simulink model "L2L_HX_test"  (R2014b)
settings: Solver=ode23tb  StartTime=0.0  StopTime=100  RelTol=1e-3
libraries: DAEMOT_Lib x9
settings Model: Creator=pangbor2  LastModifiedBy=koeln2

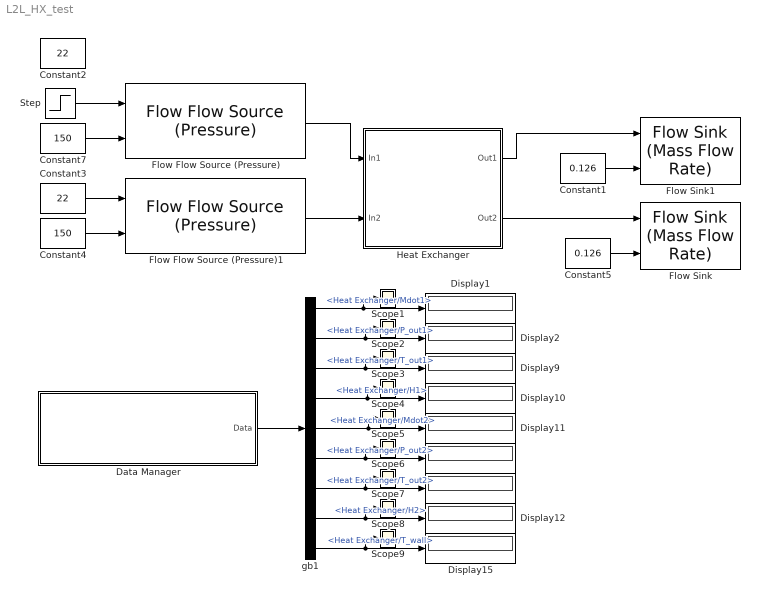
== system L2L_HX_test ==
  "  " : Display
  "   " : Display
  Constant1 : Constant  Value=0.126
  Constant2 : Constant  Value=22
  Constant3 : Constant  Value=22
  Constant4 : Constant  Value=150
  Constant5 : Constant  Value=0.126
  Constant7 : Constant  Value=150
  Data Manager : Subsystem  AncestorBlock=DAEMOT_Lib/Support Functions/Data Manager  mask{null=0}
      mask init:
      | set_param(gcb, 'LinkStatus', 'inactive')    % disable the library link
      settings: OpenFcn=data_manager
      mask Display: str ='Heat Exchanger/Mdot1\nHeat Exchanger/P_out1\nHeat Exchanger/T_out1\nHeat Exchanger/H1\nHeat Exchanger/Mdot2\nHeat Exchanger/P_out2\nHeat Exchanger/T_out2\nHeat Exchanger/H2\nHeat Exchanger/T_wall'; fprintf(str)
  Display{1..2,9..12,15} (7 alike) : Display
  Flow Flow Source (Pressure) : DAEMOT_Lib/Components/Flow Flow Source (Pressure)  M_ext=on  M=0  T_ext=on  T=0  P_ext=on  P=0
  Flow Flow Source (Pressure)1 : DAEMOT_Lib/Components/Flow Flow Source (Pressure)  M_ext=on  M=0  T_ext=on  T=0  P_ext=on  P=0
  Flow Sink : DAEMOT_Lib/Components/Flow Sink (Mass Flow Rate)  M_ext=on  M=0  T_ext=on  T=0  P_ext=on  P=0
  Flow Sink1 : DAEMOT_Lib/Components/Flow Sink (Mass Flow Rate)  M_ext=on  M=0  T_ext=on  T=0  P_ext=on  P=0
  Heat Exchanger : Subsystem  AncestorBlock=DAEMOT_Lib/Components/Heat Exchanger  mask(Heat Exchanger){Tw_init=22, fld1=PG50, P1_init=110, T1_init=22, f1=2, KL1=0, fld2=PG50, P2_init=110, T2_init=22, f2=2, KL2=0, M_wall=1, Cp_wall=0.9, Pass1=6, b1=1*1e-3, W1=87*1e-3, L1=0.193, e1=0.0015*1e-3, Nu_lam1=5.6153, Pass2=6, b2=1*1e-3, W2=87*1e-3, L2=0.193, e2=0.0015*1e-3, Nu_lam2=5.6153}
      mask prompts: Tw_init "Initial Wall Temperature [°C]"; fld1 "Fluid Type 1"; P1_init "Initial Outlet 1 Pressure [kPa]"; T1_init "Initial Outlet 1 Temperature [°C]"; f1 "Friction Factor [-]"; KL1 "Minor Losses [-]"; fld2 "Fluid Type 2"; P2_init "Initial Outlet 2 Pressure [kPa]"; T2_init "Initial Outlet 2 Temperature [°C]"; f2 "Friction Factor [-]"; KL2 "Minor Losses [-]"; M_wall "Wall Mass [kg]"; Cp_wall "Wall Specific Heat [kJ/kg*K]"; Pass1 "Number of Passes"; b1 "Plate Spacing [m]"; W1 "Plate Width [m]"; L1 "Plate Length [m]"; e1 "Surface Roughness [m] (0.0015mm for copper, 0.01mm for rubber, 0mm for plastic)"; Nu_lam1 "Laminar Nu"; Pass2 "Number of Passes"; b2 "Plate Spacing [m]"; W2 "Plate Width [m]"; L2 "Plate Length [m]"; e2 "Surface Roughness [m] (0.0015mm for copper, 0.01mm for rubber, 0mm for plastic)"; Nu_lam2 "Laminar Nu"
      mask help: Tracks the time rate of change of the pressure, wall temperature, and exit flow temperatures.
      mask init:
      | load('Fluids.mat');
      | Fluid1 = eval(['Fluid.',fld1]);
      | Fluid2 = eval(['Fluid.',fld2]);
      | 
      | load('Moody.mat');
      | 
      | load('Laminar_Props.mat')
      | Nu_lam1 = interp1(LamProps.b_a,LamProps.Nu,max(W1,b1)/min(W1,b1));
      | Nu_lam2 = interp1(LamProps.b_a,LamProps.Nu,max(W2,b2)/min(W2,b2));
      | set_param(gcb,'Nu_lam1',num2str(Nu_lam1));
      | set_param(gcb,'Nu_lam2',num2str(Nu_lam2));
      settings: OpenFcn=|
      | load('Fluids.mat');
      | Set_Fluid_Popup_Names( Fluid )
      mask TypeOptions fld1: Fuel | Water | Air | PG50
      mask TypeOptions fld2: Fuel | Water | Air | PG50
      mask DialogControl Container18 Prompt: Side 1
      mask DialogControl Container17 Prompt: Side 2
      mask DialogControl Container14 Prompt: Component Sizing - Nominal Values
      mask DialogControl Container8 Prompt: Side 1
      mask DialogControl Container9 Prompt: Side 2
      mask Display:
      | image(imread('HX.jpg'))
      | 
      | text(0.5,0.95,['{\bf ',fld1,'/',fld2,' HX}'],'TexMode','on','horizontalAlignment', 'center')
      | text(0.5,0.08,['{-----(P)}'],'TexMode','on','horizontalAlignment', 'center')
      | 
      | port_label('input',1,['In 1 (',fld1,')'])
      | port_label('input',2,['In 2 (',fld2,')'])
      | port_label('output',1,['Out 1 (',fld1,')'])
      | port_label('output',2,['Out 2 (',fld2,')'])
  Scope{1..9} (9 alike) : Scope
      Scope3 settings: SaveName=ScopeData2
      Scope4 settings: SaveName=ScopeData3
      Scope5 settings: SaveName=ScopeData4
      Scope6 settings: SaveName=ScopeData5
      Scope7 settings: SaveName=ScopeData6
      Scope8 settings: SaveName=ScopeData7
      Scope9 settings: SaveName=ScopeData8
  Step : Step  Time=20  Before=22  After=50  SampleTime=0
  gb1 : BusSelector  OutputSignals=Heat Exchanger/Mdot1,Heat Exchanger/P_out1,Heat Exchanger/T_out1,Heat Exchanger/H1,Heat Exchanger/Mdot2,Heat Exchanger/P_out2,Heat Exchanger/T_out2,Heat Exchanger/H2,Heat Exchanger/T_wall
  wires:
  Constant5/1 -> Flow Sink/2
  Heat Exchanger/2(Out2) -> Flow Sink/1
  Constant1/1 -> Flow Sink1/2
  Heat Exchanger/1(Out1) -> Flow Sink1/1
  Flow Flow Source (Pressure)/1 -> Heat Exchanger/1(In1)
  Flow Flow Source (Pressure)1/1 -> Heat Exchanger/2(In2)
  Constant7/1 -> Flow Flow Source (Pressure)/2
  Step/1 -> Flow Flow Source (Pressure)/1
  Constant4/1 -> Flow Flow Source (Pressure)1/2
  Constant3/1 -> Flow Flow Source (Pressure)1/1
  Data Manager/1(Data) -> gb1/1
  gb1/1 -> Scope1/1, Display1/1  "<Heat Exchanger/Mdot1>"
  gb1/2 -> Display2/1, Scope2/1  "<Heat Exchanger/P_out1>"
  gb1/3 -> Display9/1, Scope3/1  "<Heat Exchanger/T_out1>"
  gb1/4 -> Scope4/1, Display10/1  "<Heat Exchanger/H1>"
  gb1/5 -> Scope5/1, Display11/1  "<Heat Exchanger/Mdot2>"
  gb1/6 -> "  "/1, Scope6/1  "<Heat Exchanger/P_out2>"
  gb1/7 -> "   "/1, Scope7/1  "<Heat Exchanger/T_out2>"
  gb1/8 -> Display12/1, Scope8/1  "<Heat Exchanger/H2>"
  gb1/9 -> Display15/1, Scope9/1  "<Heat Exchanger/T_wall>"

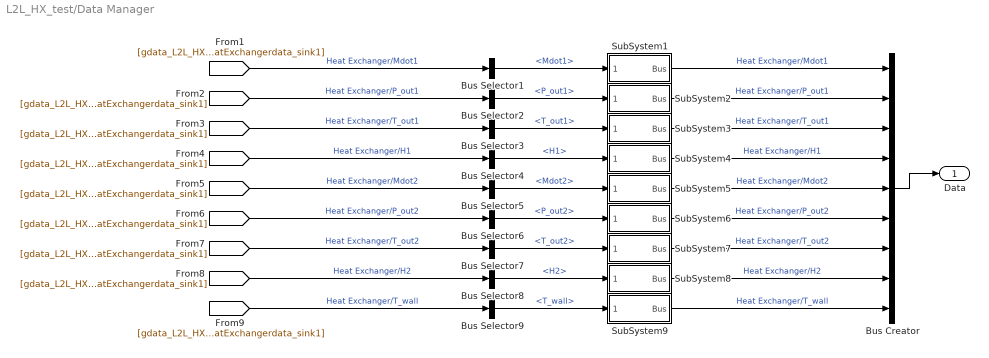
== system L2L_HX_test/Data Manager ==
  Bus Creator : BusCreator  Inputs=9
  Bus Selector1 : BusSelector  OutputSignals=Mdot1
  Bus Selector2 : BusSelector  OutputSignals=P_out1
  Bus Selector3 : BusSelector  OutputSignals=T_out1
  Bus Selector4 : BusSelector  OutputSignals=H1
  Bus Selector5 : BusSelector  OutputSignals=Mdot2
  Bus Selector6 : BusSelector  OutputSignals=P_out2
  Bus Selector7 : BusSelector  OutputSignals=T_out2
  Bus Selector8 : BusSelector  OutputSignals=H2
  Bus Selector9 : BusSelector  OutputSignals=T_wall
  SubSystem1 : Subsystem
  SubSystem2 : Subsystem
  SubSystem3 : Subsystem
  SubSystem4 : Subsystem
  SubSystem5 : Subsystem
  SubSystem6 : Subsystem
  SubSystem7 : Subsystem
  SubSystem8 : Subsystem
  SubSystem9 : Subsystem
  Data : Outport
  wires:
  Bus Creator/1 -> Data/1
  [gdata_L2L_HX_testHeatExchangerdata_sink1] -> Bus Selector1/1  "Heat Exchanger/Mdot1"
  Bus Selector1/1 -> SubSystem1/1(Rename)  "<Mdot1>"
  SubSystem1/1(Bus) -> Bus Creator/1  "Heat Exchanger/Mdot1"
  [gdata_L2L_HX_testHeatExchangerdata_sink1] -> Bus Selector2/1  "Heat Exchanger/P_out1"
  Bus Selector2/1 -> SubSystem2/1(Rename)  "<P_out1>"
  SubSystem2/1(Bus) -> Bus Creator/2  "Heat Exchanger/P_out1"
  [gdata_L2L_HX_testHeatExchangerdata_sink1] -> Bus Selector3/1  "Heat Exchanger/T_out1"
  Bus Selector3/1 -> SubSystem3/1(Rename)  "<T_out1>"
  SubSystem3/1(Bus) -> Bus Creator/3  "Heat Exchanger/T_out1"
  [gdata_L2L_HX_testHeatExchangerdata_sink1] -> Bus Selector4/1  "Heat Exchanger/H1"
  Bus Selector4/1 -> SubSystem4/1(Rename)  "<H1>"
  SubSystem4/1(Bus) -> Bus Creator/4  "Heat Exchanger/H1"
  [gdata_L2L_HX_testHeatExchangerdata_sink1] -> Bus Selector5/1  "Heat Exchanger/Mdot2"
  Bus Selector5/1 -> SubSystem5/1(Rename)  "<Mdot2>"
  SubSystem5/1(Bus) -> Bus Creator/5  "Heat Exchanger/Mdot2"
  [gdata_L2L_HX_testHeatExchangerdata_sink1] -> Bus Selector6/1  "Heat Exchanger/P_out2"
  Bus Selector6/1 -> SubSystem6/1(Rename)  "<P_out2>"
  SubSystem6/1(Bus) -> Bus Creator/6  "Heat Exchanger/P_out2"
  [gdata_L2L_HX_testHeatExchangerdata_sink1] -> Bus Selector7/1  "Heat Exchanger/T_out2"
  Bus Selector7/1 -> SubSystem7/1(Rename)  "<T_out2>"
  SubSystem7/1(Bus) -> Bus Creator/7  "Heat Exchanger/T_out2"
  [gdata_L2L_HX_testHeatExchangerdata_sink1] -> Bus Selector8/1  "Heat Exchanger/H2"
  Bus Selector8/1 -> SubSystem8/1(Rename)  "<H2>"
  SubSystem8/1(Bus) -> Bus Creator/8  "Heat Exchanger/H2"
  [gdata_L2L_HX_testHeatExchangerdata_sink1] -> Bus Selector9/1  "Heat Exchanger/T_wall"
  Bus Selector9/1 -> SubSystem9/1(Rename)  "<T_wall>"
  SubSystem9/1(Bus) -> Bus Creator/9  "Heat Exchanger/T_wall"

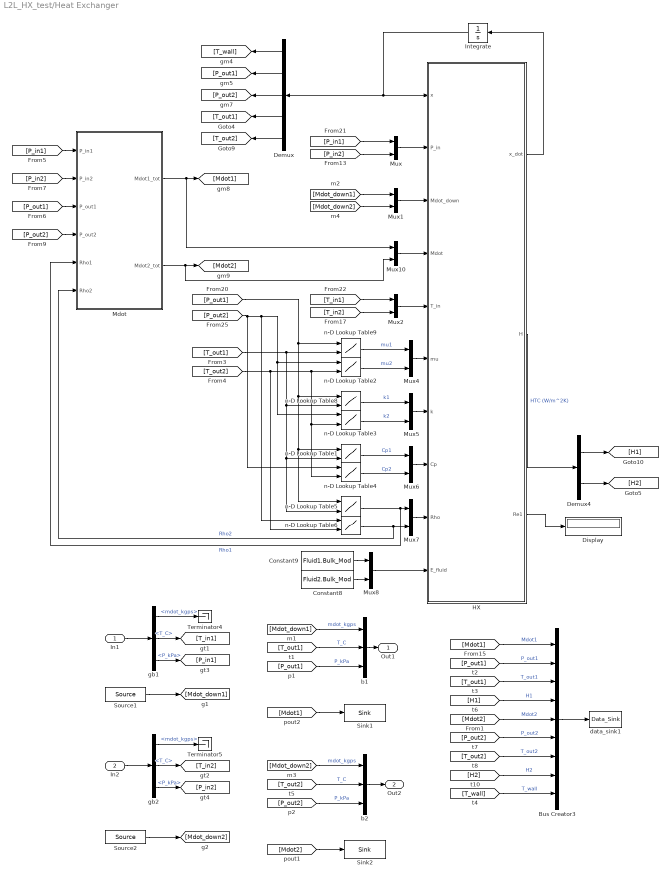
== system L2L_HX_test/Heat Exchanger ==
  In1 : Inport
  In2 : Inport  Port=2
  Bus Creator3 : BusCreator  Inputs=9
  Constant8 : Constant  Value=Fluid2.Bulk_Mod
  Constant9 : Constant  Value=Fluid1.Bulk_Mod
  Demux : Demux  Outputs=5
  Demux4 : Demux  Outputs=2
  Display : Display
  HX : MATLAB Function  TreatAsAtomicUnit=on
  Integrate : Integrator  InitialCondition=[Tw_init P1_init P2_init T1_init T2_init]
  Mdot : MATLAB Function  TreatAsAtomicUnit=on
  Mux{,1..2,4..8,10} (9 alike) : Mux  Inputs=2
  Sink1 : DAEMOT_Lib/Support Functions/Sink
  Sink2 : DAEMOT_Lib/Support Functions/Sink
  Source1 : DAEMOT_Lib/Support Functions/Source
  Source2 : DAEMOT_Lib/Support Functions/Source
  Terminator4 : Terminator
  Terminator5 : Terminator
  b1 : BusCreator  Inputs=3
  b2 : BusCreator  Inputs=3
  data_sink1 : DAEMOT_Lib/Support Functions/Data_Sink
  gb1 : BusSelector  OutputSignals=mdot_kgps,T_C,P_kPa
  gb2 : BusSelector  OutputSignals=mdot_kgps,T_C,P_kPa
  n-D Lookup Table1 : Lookup_n-D  BreakpointsForDimension1=Fluid1.P  BreakpointsForDimension2=Fluid1.T  BreakpointsForDimension3=[5, 7]  Table=Fluid1.C_pt  ExtrapMethod=Clip  RndMeth=Simplest  InputSameDT=on
  n-D Lookup Table2 : Lookup_n-D  BreakpointsForDimension1=Fluid2.P  BreakpointsForDimension2=Fluid2.T  BreakpointsForDimension3=[5, 7]  Table=Fluid2.Mu_pt  ExtrapMethod=Clip  UseLastTableValue=on  RndMeth=Simplest  InputSameDT=on
  n-D Lookup Table3 : Lookup_n-D  BreakpointsForDimension1=Fluid2.P  BreakpointsForDimension2=Fluid2.T  BreakpointsForDimension3=[5, 7]  Table=Fluid2.K_pt  ExtrapMethod=Clip  UseLastTableValue=on  RndMeth=Simplest  InputSameDT=on
  n-D Lookup Table4 : Lookup_n-D  BreakpointsForDimension1=Fluid2.P  BreakpointsForDimension2=Fluid2.T  BreakpointsForDimension3=[5, 7]  Table=Fluid2.C_pt  ExtrapMethod=Clip  UseLastTableValue=on  RndMeth=Simplest  InputSameDT=on
  n-D Lookup Table5 : Lookup_n-D  BreakpointsForDimension1=Fluid1.P  BreakpointsForDimension2=Fluid1.T  BreakpointsForDimension3=[5, 7]  Table=Fluid1.Rho_pt  ExtrapMethod=Clip  UseLastTableValue=on  RndMeth=Simplest  InputSameDT=on
  n-D Lookup Table6 : Lookup_n-D  BreakpointsForDimension1=Fluid2.P  BreakpointsForDimension2=Fluid2.T  BreakpointsForDimension3=[5, 7]  Table=Fluid2.Rho_pt  ExtrapMethod=Clip  UseLastTableValue=on  RndMeth=Simplest  InputSameDT=on
  n-D Lookup Table8 : Lookup_n-D  BreakpointsForDimension1=Fluid1.P  BreakpointsForDimension2=Fluid1.T  BreakpointsForDimension3=[5, 7]  Table=Fluid1.K_pt  ExtrapMethod=Clip  UseLastTableValue=on  RndMeth=Simplest  InputSameDT=on
  n-D Lookup Table9 : Lookup_n-D  BreakpointsForDimension1=Fluid1.P  BreakpointsForDimension2=Fluid1.T  BreakpointsForDimension3=[5, 7]  Table=Fluid1.Mu_pt  ExtrapMethod=Clip  UseLastTableValue=on  RndMeth=Simplest  InputSameDT=on
  Out1 : Outport
  Out2 : Outport  Port=2
  wires:
  b1/1 -> Out1/1
  [Mdot_down1] -> b1/1  "mdot_kgps"
  gb1/2 -> [T_in1]  "<T_C>"
  [T_out1] -> b1/2  "T_C"
  gb1/1 -> Terminator4/1  "<mdot_kgps>"
  In1/1 -> gb1/1
  [P_out1] -> b1/3  "P_kPa"
  gb1/3 -> [P_in1]  "<P_kPa>"
  [Mdot1] -> Sink1/1
  [P_in1] -> Mux/1
  Source1/1 -> [Mdot_down1]
  [Mdot_down1] -> Mux1/1
  [T_in1] -> Mux2/1
  HX/1(x_dot) -> Integrate/1
  Integrate/1 -> HX/1(x), Demux/1
  Demux/1 -> [T_wall]
  Demux/2 -> [P_out1]
  HX/2(H) -> Demux4/1  "HTC (W/m^2K)"
  n-D Lookup Table8/1 -> Mux5/1  "k1"
  n-D Lookup Table9/1 -> Mux4/1  "mu1"
  [T_out1] -> n-D Lookup Table9/2, n-D Lookup Table5/2, n-D Lookup Table1/2, n-D Lookup Table8/2
  [P_out1] -> n-D Lookup Table5/1, n-D Lookup Table1/1, n-D Lookup Table8/1, n-D Lookup Table9/1
  n-D Lookup Table1/1 -> Mux6/1  "Cp1"
  n-D Lookup Table5/1 -> Mdot/5(Rho1), Mux7/1  "Rho1"
  gb2/2 -> [T_in2]  "<T_C>"
  gb2/1 -> Terminator5/1  "<mdot_kgps>"
  In2/1 -> gb2/1
  gb2/3 -> [P_in2]  "<P_kPa>"
  Source2/1 -> [Mdot_down2]
  b2/1 -> Out2/1
  [Mdot_down2] -> b2/1  "mdot_kgps"
  [T_out2] -> b2/2  "T_C"
  [P_out2] -> b2/3  "P_kPa"
  [Mdot2] -> Sink2/1
  Mux/1 -> HX/2(P_in)
  [P_in2] -> Mux/2
  Mux1/1 -> HX/3(Mdot_down)
  [Mdot_down2] -> Mux1/2
  Mux2/1 -> HX/5(T_in)
  [T_in2] -> Mux2/2
  Mux4/1 -> HX/6(mu)
  n-D Lookup Table2/1 -> Mux4/2  "mu2"
  [P_out2] -> n-D Lookup Table4/1, n-D Lookup Table6/1, n-D Lookup Table3/1, n-D Lookup Table2/1
  [T_out2] -> n-D Lookup Table3/2, n-D Lookup Table4/2, n-D Lookup Table2/2, n-D Lookup Table6/2
  Mux5/1 -> HX/7(k)
  n-D Lookup Table3/1 -> Mux5/2  "k2"
  Mux6/1 -> HX/8(Cp)
  n-D Lookup Table4/1 -> Mux6/2  "Cp2"
  Mux7/1 -> HX/9(Rho)
  Mux8/1 -> HX/10(E_fluid)
  Demux4/1 -> [H1]
  Demux4/2 -> [H2]
  Demux/3 -> [P_out2]
  Constant9/1 -> Mux8/1
  Constant8/1 -> Mux8/2
  [H2] -> Bus Creator3/8  "H2"
  [T_out2] -> Bus Creator3/7  "T_out2"
  [P_out2] -> Bus Creator3/6  "P_out2"
  [Mdot2] -> Bus Creator3/5  "Mdot2"
  [H1] -> Bus Creator3/4  "H1"
  [T_out1] -> Bus Creator3/3  "T_out1"
  [T_wall] -> Bus Creator3/9  "T_wall"
  [P_out1] -> Bus Creator3/2  "P_out1"
  [Mdot1] -> Bus Creator3/1  "Mdot1"
  Bus Creator3/1 -> data_sink1/1
  [P_in1] -> Mdot/1(P_in1)
  n-D Lookup Table6/1 -> Mdot/6(Rho2), Mux7/2  "Rho2"
  [P_in2] -> Mdot/2(P_in2)
  [P_out2] -> Mdot/4(P_out2)
  Demux/4 -> [T_out1]
  Demux/5 -> [T_out2]
  Mdot/1(Mdot1_tot) -> Mux10/1, [Mdot1]
  Mux10/1 -> HX/4(Mdot)
  Mdot/2(Mdot2_tot) -> Mux10/2, [Mdot2]
  [P_out1] -> Mdot/3(P_out1)
  HX/3(Re1) -> Display/1

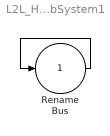
== system L2L_HX_test/Data Manager/SubSystem1 ==
  Rename : Inport
  Bus : Outport
  wires:
  Rename/1 -> Bus/1

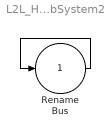
== system L2L_HX_test/Data Manager/SubSystem2 ==
  Rename : Inport
  Bus : Outport
  wires:
  Rename/1 -> Bus/1

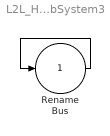
== system L2L_HX_test/Data Manager/SubSystem3 ==
  Rename : Inport
  Bus : Outport
  wires:
  Rename/1 -> Bus/1

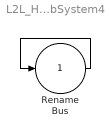
== system L2L_HX_test/Data Manager/SubSystem4 ==
  Rename : Inport
  Bus : Outport
  wires:
  Rename/1 -> Bus/1

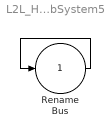
== system L2L_HX_test/Data Manager/SubSystem5 ==
  Rename : Inport
  Bus : Outport
  wires:
  Rename/1 -> Bus/1

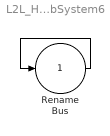
== system L2L_HX_test/Data Manager/SubSystem6 ==
  Rename : Inport
  Bus : Outport
  wires:
  Rename/1 -> Bus/1

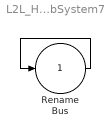
== system L2L_HX_test/Data Manager/SubSystem7 ==
  Rename : Inport
  Bus : Outport
  wires:
  Rename/1 -> Bus/1

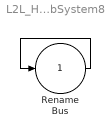
== system L2L_HX_test/Data Manager/SubSystem8 ==
  Rename : Inport
  Bus : Outport
  wires:
  Rename/1 -> Bus/1

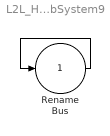
== system L2L_HX_test/Data Manager/SubSystem9 ==
  Rename : Inport
  Bus : Outport
  wires:
  Rename/1 -> Bus/1

== matlab function L2L_HX_test/Heat Exchanger/HX ==
  data: x input; x_dot output; P_in input size=2; Mdot_down input size=2; Mdot input; T_in input size=2; H output; mu input size=2; k input size=2; Cp input size=2; Rho input size=2; E_fluid input size=2; M_wall parameter; Cp_wall parameter; Pass1 parameter; Pass2 parameter; f1 parameter; f2 parameter; KL1 parameter; KL2 parameter; b1 parameter; b2 parameter; W1 parameter; W2 parameter; L1 parameter; L2 parameter; Nu_lam1 parameter; Nu_lam2 parameter; Re1 output
function [x_dot,H,Re1]  = HX(x,P_in,Mdot_down,Mdot,T_in,mu,k,Cp,Rho,E_fluid,M_wall,Cp_wall,Pass1,Pass2,f1,f2,KL1,KL2,b1,b2,W1,W2,L1,L2,Nu_lam1,Nu_lam2)

% Parse data
P_in1       = P_in(1);
P_in2       = P_in(2);
Mdot_down1  = Mdot_down(1);
Mdot_down2  = Mdot_down(2);
Mdot1       = Mdot(1);
Mdot2       = Mdot(2);
T_in1       = T_in(1);
T_in2       = T_in(2);
mu1         = mu(1);
mu2         = mu(2);
k1          = k(1);
k2          = k(2);
Cp1         = Cp(1);
Cp2         = Cp(2);
Rho1        = Rho(1);
Rho2        = Rho(2);
E_fluid1    = E_fluid(1);
E_fluid2    = E_fluid(2);

% Constants and Conversions
Mdot_down1_pass = Mdot_down1/Pass1;
Mdot_down2_pass = Mdot_down2/Pass2;
Mdot1_pass = Mdot1/Pass1;
Mdot2_pass = Mdot2/Pass2;
A_ht1    = L1*(2*b1+2*W1);         % Heat transfer area
A_ht2    = L2*(2*b2+2*W2);         % Heat transfer area
V1       = L1*b1*W1;               % Volume per pass
V2       = L2*b2*W2;               % Volume per pass
Cp1      = 1000*Cp1;               % Convert Cp from J/g*K to J/kg*K
Cp2      = 1000*Cp2;               % Convert Cp from J/g*K to J/kg*K
k1       = 1000*k1;                % Convert k from kW/m*K to W/m*K
k2       = 1000*k2;                % Convert k from kW/m*K to W/m*K
C_wall   = M_wall*Cp_wall;         % Heat Capacitance (kJ/K)
C_wall   = 1000*C_wall;            % Covnert heat capacitance from kJ/K to J/K
D1       = 4*b1*W1/(2*b1+2*W1);    % Hydraulic diameter (side 1) (see Incropera, Eq. 8.66)
D2       = 4*b2*W2/(2*b2+2*W2);    % Hydraulic diameter (side 2) (see Incropera, Eq. 8.66)

% Parse states
Tw      = x(1);                 % Wall temperature
P1      = x(2);                 % Outlet pressure (side 1)
P2      = x(3);                 % Outlet pressure (side 2)
T1      = x(4);                 % Outlet temperature (side 1)
T2      = x(5);                 % Outlet temperature (side 2)

% Additional intermediate variable calculations
dP1         = (P_in1-P1)*1000;  % Pressure differential (side 1) [Pa]
dP2         = (P_in2-P2)*1000;  % Pressure differential (side 2) [Pa]
um1         = sign(dP1)*sqrt(2*abs(dP1)/(Rho1*(f1*L1/D1+KL1)));   % Fluid velocity (side 1) [m/s]
um2         = sign(dP2)*sqrt(2*abs(dP2)/(Rho2*(f2*L2/D2+KL2)));   % Fluid velocity (side 2) [m/s]
Re1         = Rho1*um1*D1/mu1;      % Reynolds number (side 1)
Re2         = Rho2*um2*D2/mu2;      % Reynolds number (side 1)
Pr1         = Cp1*mu1/k1;           % Prandtl number (side 1) (see Incropera, Table 6.2)
Pr2         = Cp2*mu2/k2;           % Prandtl number (side 2) (see Incropera, Table 6.2)
if Re1 < 2300
    Nu1 = Nu_lam1; % (inteprolated from Incropera, Table 8.1 in initialization)
else
    Nu1 = (f1/8)*(Re1-1000)*Pr1 / (1+12.7*(f1/8)^.5*(Pr1^(2/3)-1)); % (see Incropera, Eq. 8.62)
end
if Re2 < 2300
    Nu2 = Nu_lam2; % (inteprolated from Incropera, Table 8.1 in initialization)
else
    Nu2 = (f2/8)*(Re2-1000)*Pr2 / (1+12.7*(f2/8)^.5*(Pr2^(2/3)-1)); % (see Incropera, Eq. 8.62)
end

% Calculate outputs
H1      = Nu1*k1/D1;        % Heat transfer coefficient (see Incropera, Table 6.2)
H2      = Nu2*k2/D2;        % Heat transfer coefficient (see Incropera, Table 6.2)
H       = [H1 H2];

% Calculate state derivatives
Tw_dot = ( H1*A_ht1*(T1-Tw) + H2*A_ht2*(T2-Tw) )/C_wall;    % Wall temperature
P1_dot = (Mdot1_pass-Mdot_down1_pass)/(V1*Rho1/E_fluid1);   % Outlet pressure (side 1)
P2_dot = (Mdot2_pass-Mdot_down2_pass)/(V2*Rho2/E_fluid2);   % Outlet pressure (side 2)
Tout1_dot = (Mdot1_pass*(T_in1-T1)+H1*A_ht1/Cp1*(Tw-T1))/(V1*Rho1);   % Outlet temperature (side 1)
Tout2_dot = (Mdot2_pass*(T_in2-T2)+H2*A_ht2/Cp2*(Tw-T2))/(V2*Rho2);   % Outlet temperature (side 2)

% Mux state derivatives
x_dot  = [Tw_dot,P1_dot,P2_dot,Tout1_dot,Tout2_dot];

end

== matlab function L2L_HX_test/Heat Exchanger/Mdot ==
  data: P_in1 input; P_in2 input; Mdot1_tot output; P_out1 input; P_out2 input; Rho1 input; Rho2 input; f1 parameter; f2 parameter; b1 parameter; b2 parameter; W1 parameter; W2 parameter; L1 parameter; L2 parameter; KL1 parameter; KL2 parameter; Mdot2_tot output; Pass1 parameter; Pass2 parameter
function [Mdot1_tot,Mdot2_tot]   = Mdot(P_in1,P_in2,P_out1,P_out2,Rho1,Rho2,f1,f2,b1,b2,W1,W2,L1,L2,KL1,KL2,Pass1,Pass2)

% Constants and Conversions
D1 = 4*b1*W1/(2*b1+2*W1);           % (see Incropera, Eq. 8.66)
D2 = 4*b2*W2/(2*b2+2*W2);           % (see Incropera, Eq. 8.66)
dP1         = (P_in1-P_out1)*1000;  % Pressure differential (side 1) [Pa]
dP2         = (P_in2-P_out2)*1000;  % Pressure differential (side 2) [Pa]
um1         = sign(dP1)*sqrt(2*abs(dP1)/(Rho1*(f1*L1/D1+KL1))); % Fluid velocity (side 1) [m/s]
um2         = sign(dP2)*sqrt(2*abs(dP2)/(Rho2*(f2*L2/D2+KL2))); % Fluid velocity (side 2) [m/s]
Mdot1_pass  = um1*Rho1*b1*W1;       % Mass flow rate per pass (side 1) [kg/s]
Mdot2_pass  = um2*Rho2*b2*W2;       % Mass flow rate per pass (side 2) [kg/s]

% Calculate outputs
Mdot1_tot = Mdot1_pass*Pass1;       % Total mass flow rate (side 1) [kg/s]
Mdot2_tot = Mdot2_pass*Pass2;       % Total mass flow rate (side 2) [kg/s]

end
